simulink model "TransferFunctionModel_trial"  (R2021a)
settings: Solver=VariableStepAuto  StartTime=0.0  StopTime=sim_time  MaxStep=0.01  RelTol=1e-3
values from neighbouring files (symbols this model uses):
  b = 3.5077E-6    (= 3.5077e-06)    [DCMotor_reduction_run.m]    (also in DCMotor_run.m; MassSpringDamper_run.m = 2; PID_ScriptOnly.m = 50; PID_SpringDamper_run.m = 10)
  F = 1    [MassSpringDamper_run.m]    (also in PID_SpringDamper_run.m = 10; TrainSimulation_run.m; TransferFunctionModel_run.m = 10)
  k = 20    [MassSpringDamper_run.m]    (also in PID_SpringDamper_run.m; PID_block_run.m; TrainSimulation_run.m = 1; TransferFunctionModel_run.m)
  M = 1    [MassSpringDamper_run.m]    (also in PID_SpringDamper_run.m; PID_block_run.m; PID_vehicle_run.m; TransferFunctionModel_run.m)
libraries: dspsrcs4 x1
settings Model: Creator=shinyh  LastModifiedBy=shinyh

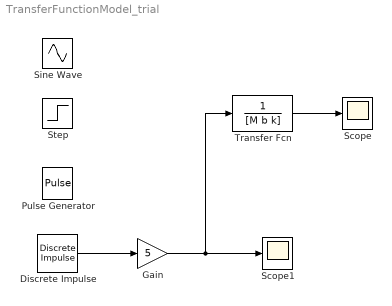
== system TransferFunctionModel_trial ==
  Discrete Impulse : dspsrcs4/Discrete  Impulse  Delay=0  SampleTime=1  FrameSample=1  OutputFrames=off  dataType=double  isSigned=on  wordLen=16  udDataType=sfix(16)  fracBitsMode=Best precision  numFracBits=15  OutDataTypeStr=double  LastOutDataTypeStr=double
  Gain : Gain  Gain=5
  Pulse Generator : DiscretePulseGenerator  PulseType=Time based  Amplitude=F  Period=10  PulseWidth=5
  Scope : Scope
  Scope1 : Scope
  Sine Wave : Sin  Amplitude=F  SampleTime=0
  Step : Step  Time=F  After=F  SampleTime=0
  Transfer Fcn : TransferFcn  Denominator=[M b k]
  wires:
  Transfer Fcn/1 -> Scope/1
  Discrete Impulse/1 -> Gain/1
  Gain/1 -> Transfer Fcn/1, Scope1/1
